simulink model "Final_System"  (R2016a)
settings: Solver=ode45  SolverMode=SingleTasking  StartTime=0.0  StopTime=8  RelTol=1e-3
settings Model: ExtModeTrigDuration=5000  Creator=yifu.wang  LastModifiedBy=yifuw
settings DataIOCC: LimitDataPoints=on  SaveFormat=Array  SignalLoggingSaveFormat=ModelDataLogs
settings OptimizationCC: BlockReduction=off  BooleanDataType=off  ExpressionDepthLimit=2147483647
settings DebuggingCC: SaveWithParameterizedLinksMsg=none  UnderspecifiedInitializationDetection=Classic  MergeDetectMultiDrivingBlocksExec=none  SignalResolutionControl=TryResolveAllWithWarning  MultiTaskDSMMsg=warning  MultiTaskCondExecSysMsg=none  StateNameClashWarn=warning
settings HardwareCC: ProdBitPerPointer=32  ProdLargestAtomicFloat=None  ProdIntDivRoundTo=Undefined  ProdEndianess=Unspecified  ProdWordSize=32  ProdHWDeviceType=32-bit Generic  TargetUnknown=on
settings ModelReferenceCC: PropagateSignalLabelsOutOfModel=off
settings ConfigComp: CovModelRefEnable=Off

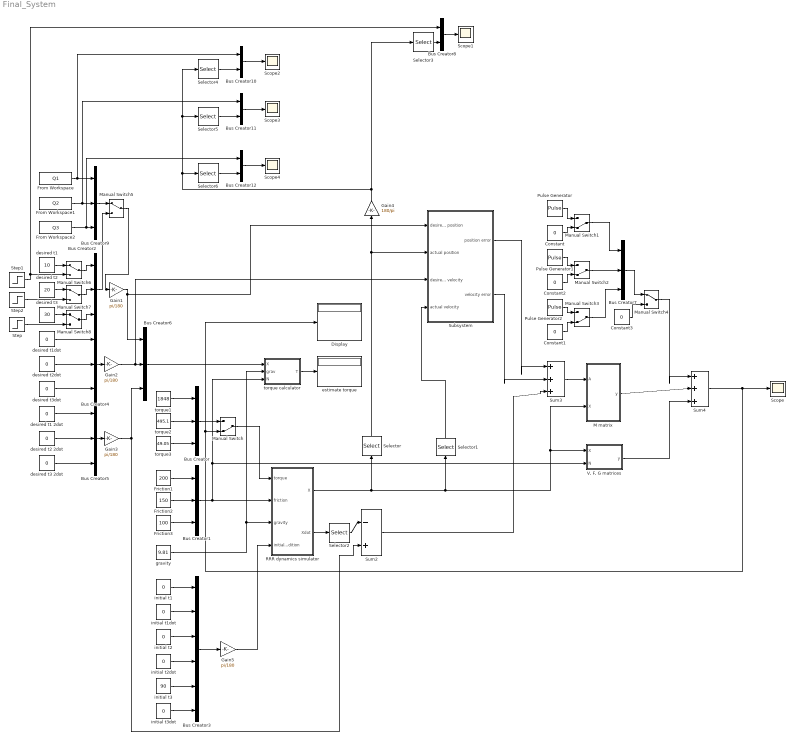
== system Final_System ==
  Bus Creator{,1..2,4..7,9} (8 alike) : BusCreator  Inputs=3
  Bus Creator{8,10..12} (4 alike) : BusCreator  Inputs=2
  Bus Creator3 : BusCreator  Inputs=6
  Constant{,1..3} (4 alike) : Constant  Value=0
  Display : Display
      settings: Decimation=3
  Friction1 : Constant  Value=200
  Friction2 : Constant  Value=150
  Friction3 : Constant  Value=100
  From Workspace : FromWorkspace  VariableName=Q1  SampleTime=0
  From Workspace1 : FromWorkspace  VariableName=Q2  SampleTime=0
  From Workspace2 : FromWorkspace  VariableName=Q3  SampleTime=0
  Gain{1..3,5} (4 alike) : Gain  Gain=pi/180
  Gain4 : Gain  Gain=180/pi
  M matrix : MATLAB Function  TreatAsAtomicUnit=on
  Manual Switch{,1..3} (4 alike) : ManualSwitch  CurrentSetting=0
  Manual Switch{4..8} (5 alike) : ManualSwitch
  Pulse Generator : DiscretePulseGenerator  PulseType=Time based  Amplitude=10  Period=10  PulseWidth=5
  Pulse Generator1 : DiscretePulseGenerator  PulseType=Time based  Amplitude=10  Period=10  PulseWidth=5
  Pulse Generator2 : DiscretePulseGenerator  PulseType=Time based  Amplitude=10  Period=10  PulseWidth=5
  RRR dynamics simulator : Subsystem
  Scope{,1..4} (5 alike) : Scope
  Selector : Selector  InputPortWidth=6  IndexOptions=Index vector (dialog)  Indices=[1 3 5]  OutputSizes=1
  Selector1 : Selector  InputPortWidth=6  IndexOptions=Index vector (dialog)  Indices=[2 4 6]  OutputSizes=1
  Selector2 : Selector  InputPortWidth=6  IndexOptions=Index vector (dialog)  Indices=[2 4 6]  OutputSizes=1
  Selector3 : Selector  InputPortWidth=3  IndexOptions=Index vector (dialog)  Indices=[3]  OutputSizes=1
  Selector4 : Selector  InputPortWidth=3  IndexOptions=Index vector (dialog)  Indices=[1]  OutputSizes=1
  Selector5 : Selector  InputPortWidth=3  IndexOptions=Index vector (dialog)  Indices=[2]  OutputSizes=1
  Selector6 : Selector  InputPortWidth=3  IndexOptions=Index vector (dialog)  Indices=[3]  OutputSizes=1
  Step : Step  SampleTime=0
  Step1 : Step  SampleTime=0
  Step2 : Step  SampleTime=0
  Subsystem : Subsystem
  Sum2 : Sum  Inputs=|-+
  Sum3 : Sum  Inputs=|+++
  Sum4 : Sum  Inputs=|+++
  "V, F, G matrices" : MATLAB Function  TreatAsAtomicUnit=on
  desired t1 : Constant  Value=10
  desired t1 2dot : Constant  Value=0
  desired t1dot : Constant  Value=0
  desired t2 : Constant  Value=20
  desired t2 2dot : Constant  Value=0
  desired t2dot : Constant  Value=0
  desired t3 : Constant  Value=30
  desired t3 2dot : Constant  Value=0
  desired t3dot : Constant  Value=0
  estimate torque : Display
      settings: Decimation=3
  gravity : Constant  Value=9.81
  initial t1 : Constant  Value=0
  initial t1dot : Constant  Value=0
  initial t2 : Constant  Value=0
  initial t2dot : Constant  Value=0
  initial t3 : Constant  Value=90
  initial t3dot : Constant  Value=0
  torque calculator : MATLAB Function  TreatAsAtomicUnit=on
  torque1 : Constant  Value=1848
  torque2 : Constant  Value=495.1
  torque3 : Constant  Value=49.05
  wires:
  gravity/1 -> RRR dynamics simulator/3(gravity), torque calculator/2(grav)
  torque1/1 -> Bus Creator/1
  torque3/1 -> Bus Creator/3
  torque2/1 -> Bus Creator/2
  Friction1/1 -> Bus Creator1/1
  Friction3/1 -> Bus Creator1/3
  Friction2/1 -> Bus Creator1/2
  torque calculator/1(T) -> estimate torque/1
  Bus Creator1/1 -> torque calculator/3(N), "V, F, G matrices"/2(N), RRR dynamics simulator/2(friction)
  Bus Creator6/1 -> torque calculator/1(X)
  initial t1/1 -> Bus Creator3/1
  initial t1dot/1 -> Bus Creator3/2
  initial t2/1 -> Bus Creator3/3
  initial t2dot/1 -> Bus Creator3/4
  initial t3/1 -> Bus Creator3/5
  initial t3dot/1 -> Bus Creator3/6
  Bus Creator3/1 -> Gain5/1
  desired t1dot/1 -> Bus Creator4/1
  desired t2dot/1 -> Bus Creator4/2
  desired t3dot/1 -> Bus Creator4/3
  desired t1 2dot/1 -> Bus Creator5/1
  desired t2 2dot/1 -> Bus Creator5/2
  desired t3 2dot/1 -> Bus Creator5/3
  Bus Creator4/1 -> Gain2/1
  Bus Creator5/1 -> Gain3/1
  RRR dynamics simulator/1(X) -> Selector/1, Selector1/1, "V, F, G matrices"/1(X), M matrix/2(X)
  Selector/1 -> Subsystem/2(actual position), Gain4/1
  RRR dynamics simulator/2(Xdot) -> Selector2/1
  Sum2/1 -> Sum3/3
  Selector2/1 -> Sum2/1
  Sum3/1 -> M matrix/1(A)
  Bus Creator/1 -> Manual Switch/1
  Sum4/1 -> Scope/1, Display/1, Manual Switch/2
  Manual Switch/1 -> RRR dynamics simulator/1(torque)
  Pulse Generator/1 -> Manual Switch1/1
  Constant/1 -> Manual Switch1/2
  Pulse Generator1/1 -> Manual Switch2/1
  Constant2/1 -> Manual Switch2/2
  Pulse Generator2/1 -> Manual Switch3/1
  Constant1/1 -> Manual Switch3/2
  Manual Switch1/1 -> Bus Creator7/1
  Manual Switch2/1 -> Bus Creator7/2
  Manual Switch3/1 -> Bus Creator7/3
  Bus Creator7/1 -> Manual Switch4/1
  Constant3/1 -> Manual Switch4/2
  "V, F, G matrices"/1(y) -> Sum4/3
  M matrix/1(y) -> Sum4/2
  Manual Switch4/1 -> Sum4/1
  Gain1/1 -> Subsystem/1(desired position), Bus Creator6/1
  Gain2/1 -> Subsystem/3(desired velocity), Bus Creator6/2
  Gain3/1 -> Sum2/2, Bus Creator6/3
  Step1/1 -> Bus Creator8/1, Manual Switch6/2
  Selector3/1 -> Bus Creator8/2
  Bus Creator8/1 -> Scope1/1
  Bus Creator9/1 -> Manual Switch5/1
  Bus Creator2/1 -> Manual Switch5/2
  Manual Switch5/1 -> Gain1/1
  desired t1/1 -> Manual Switch6/1
  Manual Switch6/1 -> Bus Creator2/1
  desired t2/1 -> Manual Switch7/1
  Step2/1 -> Manual Switch7/2
  Manual Switch7/1 -> Bus Creator2/2
  desired t3/1 -> Manual Switch8/1
  Step/1 -> Manual Switch8/2
  Manual Switch8/1 -> Bus Creator2/3
  Gain5/1 -> RRR dynamics simulator/4(initial condition)
  Selector1/1 -> Subsystem/4(actual velocity)
  Subsystem/1(position error) -> Sum3/1
  Subsystem/2(velocity error) -> Sum3/2
  From Workspace/1 -> Bus Creator10/1, Bus Creator9/1
  From Workspace1/1 -> Bus Creator11/1, Bus Creator9/2
  From Workspace2/1 -> Bus Creator12/1, Bus Creator9/3
  Selector4/1 -> Bus Creator10/2
  Bus Creator10/1 -> Scope2/1
  Gain4/1 -> Selector4/1, Selector5/1, Selector6/1, Selector3/1
  Selector5/1 -> Bus Creator11/2
  Bus Creator11/1 -> Scope3/1
  Selector6/1 -> Bus Creator12/2
  Bus Creator12/1 -> Scope4/1

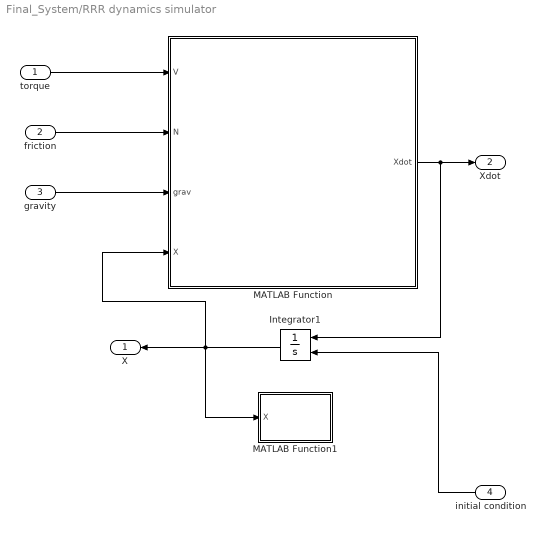
== system Final_System/RRR dynamics simulator ==
  torque : Inport
  friction : Inport  Port=2
  gravity : Inport  Port=3
  initial condition : Inport  Port=4
  Integrator1 : Integrator  InitialConditionSource=external  InitialCondition=[pi/18 0 pi/9 0 pi/6 0]
  MATLAB Function : MATLAB Function  TreatAsAtomicUnit=on
  MATLAB Function1 : MATLAB Function  TreatAsAtomicUnit=on
  X : Outport
  Xdot : Outport  Port=2
  wires:
  gravity/1 -> MATLAB Function/3(grav)
  friction/1 -> MATLAB Function/2(N)
  Integrator1/1 -> MATLAB Function/4(X), X/1, MATLAB Function1/1(X)
  MATLAB Function/1(Xdot) -> Integrator1/1, Xdot/1
  initial condition/1 -> Integrator1/2
  torque/1 -> MATLAB Function/1(V)

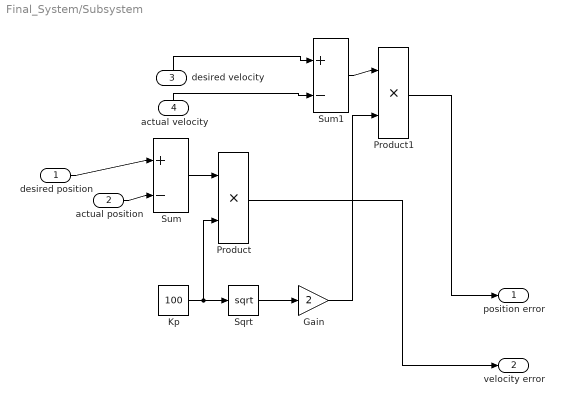
== system Final_System/Subsystem ==
  desired position : Inport
  actual position : Inport  Port=2
  desired velocity : Inport  Port=3
  actual velocity : Inport  Port=4
  Gain : Gain  Gain=2
  Kp : Constant  Value=100
  Product : Product  RndMeth=Zero
  Product1 : Product  RndMeth=Zero
  Sqrt : Sqrt  SaturateOnIntegerOverflow=on
  Sum : Sum  Inputs=|+-
  Sum1 : Sum  Inputs=|+-
  position error : Outport
  velocity error : Outport  Port=2
  wires:
  Kp/1 -> Product/2, Sqrt/1
  actual velocity/1 -> Sum1/2
  Gain/1 -> Product1/2
  Product1/1 -> position error/1
  Sum/1 -> Product/1
  Sqrt/1 -> Gain/1
  Product/1 -> velocity error/1
  Sum1/1 -> Product1/1
  actual position/1 -> Sum/2
  desired velocity/1 -> Sum1/1
  desired position/1 -> Sum/1

== matlab function Final_System/RRR dynamics simulator/MATLAB Function1 ==
  data: X input
function plot(X)

t1 = X(1,1);
t2 = X(3,1);
t3 = X(5,1);

L1 = 4;
L2 = 3;
L3 = 2;

c1 = cos(t1);
s1 = sin(t1);
c2 = cos(t2);
s2 = sin(t2);
c3 = cos(t3);
s3 = sin(t3);

T01 = [c1 -s1 0 0; s1 c1 0 0 ;0 0 1 0 ; 0 0 0 1];
T12 = [c2 -s2 0 L1; s2 c2 0 0; 0 0 1 0; 0 0 0 1];
T23 = [c3 -s3 0 L2; s3 c3 0 0; 0 0 1 0; 0 0 0 1];
T3E = [1 0 0 L3; 0 1 0 0; 0 0 1 0; 0 0 0 1];

T02 = T01 * T12;
T03 = T02 * T23;
T0E = T03 * T3E;

P1 = T01 * [L1;0;0;1];
P2 = T02 * [L2;0;0;1];
P3 = T03 * [L3;0;0;1];
P4 = T0E * [0;0.5;0;1];
P5 = T0E * [0.5;0.5;0;1];
P6 = T0E * [0;-0.5;0;1];
P7 = T0E * [0.5;-0.5;0;1];

X1 = [0 P1(1,1) P2(1,1) P3(1,1) P4(1,1) P5(1,1)];
Y1 = [0 P1(2,1) P2(2,1) P3(2,1) P4(2,1) P5(2,1)];
X2 = [P1(1,1) P2(1,1)];
Y2 = [P1(2,1) P2(2,1)];
X3 = [P2(1,1) P3(1,1) P4(1,1) P5(1,1)];
Y3 = [P2(2,1) P3(2,1) P4(2,1) P5(2,1)];
X4 =[P3(1,1) P6(1,1) P7(1,1)];
Y4 =[P3(2,1) P6(2,1) P7(2,1)];

% Z = [0 P1(3,1) P2(3,1) P3(3,1)];


%  axis1 = linspace(-5,15,200);
%  plot3(axis1*0,axis1,axis1*0,'b',axis1,axis1*0,axis1*0,'b',axis1*0,axis1*0,axis1,'b',X,Y,Z);
plot(X1,Y1,'r',X2,Y2,'b',X3,Y3,'g',X4,Y4,'g','linewidth',3);
% drawnow
%  axis([-20 20 -20 20 -20 20]);
axis([-15 15 -15 15]);
grid on;
end

== matlab function Final_System/RRR dynamics simulator/MATLAB Function ==
  data: V input; N input; Xdot output; grav input; X input
function Xdot = fcn(V,N,grav,X)
t1 = X(1);
t1dot = X(2);
t2 = X(3);
t2dot = X(4);
t3 = X(5);
t3dot = X(6);

v1 = V(1);
v2 = V(2);
v3 = V(3);

Friction1 = N(1);
Friction2 = N(2);
Friction3 = N(3);

Xdot = [0;0;0;0;0;0];
V_0 = [v1;v2;v3];

Xdot(1) = X(2);
Xdot(3) = X(4);
Xdot(5) = X(6);



M = [80*cos(t2 + t3) + 420*cos(t2) + 60*cos(t3) + 12291/20, 40*cos(t2 + t3) + 210*cos(t2) + 60*cos(t3) + 2681/20, 40*cos(t2 + t3) + 30*cos(t3) + 101/10;
     40*cos(t2 + t3) + 210*cos(t2) + 60*cos(t3) + 2681/20,                                 60*cos(t3) + 2681/20,                   30*cos(t3) + 101/10;
                    40*cos(t2 + t3) + 30*cos(t3) + 101/10,                                  30*cos(t3) + 101/10,                                101/10];

V1 = [                             0, - 40*sin(t2 + t3) - 210*sin(t2), - 40*sin(t2 + t3) - 30*sin(t3);
       40*sin(t2 + t3) + 210*sin(t2),                               0,                    -30*sin(t3);
        40*sin(t2 + t3) + 30*sin(t3),                      30*sin(t3),                              0];
    
V2 = [ - 40*sin(t2 + t3) - 210*sin(t2), - 40*sin(t2 + t3) - 30*sin(t3), - 40*sin(t2 + t3) - 30*sin(t3);
                                     0,                    -30*sin(t3),                    -30*sin(t3);
                            30*sin(t3),                              0,                              0];     
         
V = V1 * [t1dot^2;t2dot^2;t3dot^2] + 2*V2*[t1dot*t2dot;t1dot*t3dot;t2dot*t3dot];

G = [(5*grav*(4*cos(t1 + t2 + t3) + 21*cos(t1 + t2) + 56*cos(t1)))/2;
              (105*grav*cos(t1 + t2))/2 + 10*grav*cos(t1 + t2 + t3);
                                         10*grav*cos(t1 + t2 + t3)];
                                     
F = [Friction1 * t1dot;
     Friction2 * t2dot;
     Friction3 * t3dot];

A = inv(M) * (V_0 - V - G - F);


Xdot(2) = A(1);
Xdot(4) = A(2);
Xdot(6) = A(3);
end

== matlab function Final_System/torque calculator ==
  data: X input; T output; grav input; N input
function T = fcn(X,grav,N)

t1 = X(1);
t1dot = X(4);
t1dot2 = X(7);
t2 = X(2);
t2dot = X(5);
t2dot2 = X(8);
t3 = X(3);
t3dot = X(6);
t3dot2 = X(9);

Friction1 = N(1);
Friction2 = N(2);
Friction3 = N(3);

M = [80*cos(t2 + t3) + 420*cos(t2) + 60*cos(t3) + 12291/20, 40*cos(t2 + t3) + 210*cos(t2) + 60*cos(t3) + 2681/20, 40*cos(t2 + t3) + 30*cos(t3) + 101/10;
     40*cos(t2 + t3) + 210*cos(t2) + 60*cos(t3) + 2681/20,                                 60*cos(t3) + 2681/20,                   30*cos(t3) + 101/10;
                    40*cos(t2 + t3) + 30*cos(t3) + 101/10,                                  30*cos(t3) + 101/10,                                101/10];

V1 = [                             0, - 40*sin(t2 + t3) - 210*sin(t2), - 40*sin(t2 + t3) - 30*sin(t3);
       40*sin(t2 + t3) + 210*sin(t2),                               0,                    -30*sin(t3);
        40*sin(t2 + t3) + 30*sin(t3),                      30*sin(t3),                              0];
    
V2 = [ - 40*sin(t2 + t3) - 210*sin(t2), - 40*sin(t2 + t3) - 30*sin(t3), - 40*sin(t2 + t3) - 30*sin(t3);
                                     0,                    -30*sin(t3),                    -30*sin(t3);
                            30*sin(t3),                              0,                              0];     
         
V = V1 * [t1dot^2;t2dot^2;t3dot^2] + 2*V2*[t1dot*t2dot;t1dot*t3dot;t2dot*t3dot];

G = [(5*grav*(4*cos(t1 + t2 + t3) + 21*cos(t1 + t2) + 56*cos(t1)))/2;
              (105*grav*cos(t1 + t2))/2 + 10*grav*cos(t1 + t2 + t3);
                                         10*grav*cos(t1 + t2 + t3)];
                                     
F = [Friction1 * X(2);
     Friction2 * X(4);
     Friction3 * X(6)];
 
T = M * [t1dot2;t2dot2;t3dot2] + V + G + F;

== matlab function Final_System/M matrix ==
  data: A input; y output; X input
function y = fcn(A,X)
t1 = X(1);
t1dot = X(2);
t2 = X(3);
t2dot = X(4);
t3 = X(5);
t3dot = X(6);

M = [80*cos(t2 + t3) + 420*cos(t2) + 60*cos(t3) + 12291/20, 40*cos(t2 + t3) + 210*cos(t2) + 60*cos(t3) + 2681/20, 40*cos(t2 + t3) + 30*cos(t3) + 101/10;
     40*cos(t2 + t3) + 210*cos(t2) + 60*cos(t3) + 2681/20,                                 60*cos(t3) + 2681/20,                   30*cos(t3) + 101/10;
                    40*cos(t2 + t3) + 30*cos(t3) + 101/10,                                  30*cos(t3) + 101/10,                                101/10];

y = M*A;

== matlab function Final_System/V, F, G matrices ==
  data: X input; y output; N input
function y = fcn(X,N)
grav = 9.81;

t1 = X(1);
t1dot = X(2);
t2 = X(3);
t2dot = X(4);
t3 = X(5);
t3dot = X(6);

Friction1 = N(1);
Friction2 = N(2);
Friction3 = N(3);

V1 = [                             0, - 40*sin(t2 + t3) - 210*sin(t2), - 40*sin(t2 + t3) - 30*sin(t3);
       40*sin(t2 + t3) + 210*sin(t2),                               0,                    -30*sin(t3);
        40*sin(t2 + t3) + 30*sin(t3),                      30*sin(t3),                              0];
    
V2 = [ - 40*sin(t2 + t3) - 210*sin(t2), - 40*sin(t2 + t3) - 30*sin(t3), - 40*sin(t2 + t3) - 30*sin(t3);
                                     0,                    -30*sin(t3),                    -30*sin(t3);
                            30*sin(t3),                              0,                              0];     
         
V = V1 * [t1dot^2;t2dot^2;t3dot^2] + 2*V2*[t1dot*t2dot;t1dot*t3dot;t2dot*t3dot];

G = [(5*grav*(4*cos(t1 + t2 + t3) + 21*cos(t1 + t2) + 56*cos(t1)))/2;
              (105*grav*cos(t1 + t2))/2 + 10*grav*cos(t1 + t2 + t3);
                                         10*grav*cos(t1 + t2 + t3)];
                                     
F = [Friction1 * X(2);
     Friction2 * X(4);
     Friction3 * X(6)];
y = V+G+F;
